simulink model "model"  (R2022b)
settings: Solver=VariableStepAuto  StartTime=0.0  StopTime=20  RelTol=1e-3
libraries: slpidlib x3, simulink x2, fuzblock x2, mpclib x1
settings Model: Creator=philf  LastModifiedBy=philf

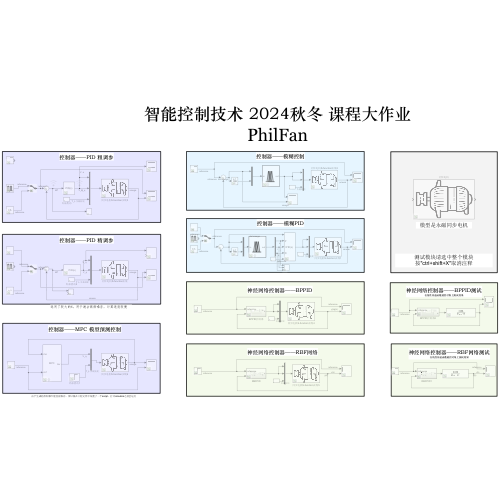
[thumbnail: Simulink's stored preview of the top-level diagram]
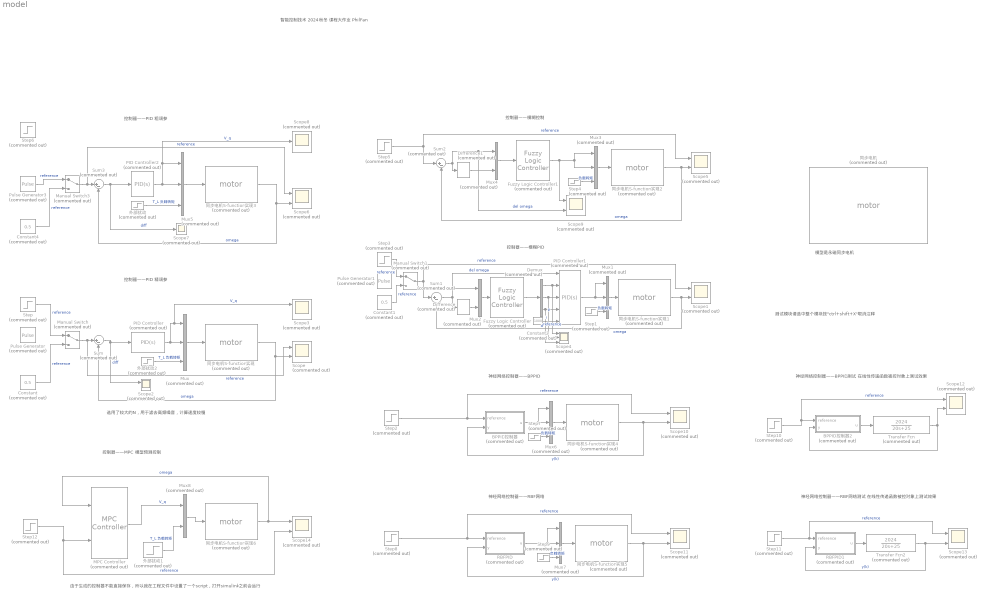
== system model ==
  note: 测试模块请选中整个模块按"ctrl+shift+X"取消注释
  note: 选用了较大的N，用于滤去高频噪音，计算速度较慢
  note: 控制器——PID 精调参
  note: 控制器——模糊PID
  note: 控制器——模糊控制
  note: 控制器——PID 粗调参
  note: 神经网络控制器——BPPID
  note: 神经网络控制器——RBF网络
  note: 神经网络控制器——BPPID测试
      | 在线性传递函数被控对象上测试效果
  note: 模型是永磁同步电机
  note: 神经网络控制器——RBF网络测试
      | 在线性传递函数被控对象上测试效果
  note: 控制器——MPC 模型预测控制
  note: 由于生成的控制器不能直接保存，所以我在工程文件中设置了一个script，打开simulink之前会运行
  note: 智能控制技术 2024秋冬 课程大作业
      | PhilFan
  BPPID控制器 : Subsystem  Commented=on
  BPPID控制器2 : Subsystem  Commented=on
  Constant : Constant  Commented=on  Value=0.5
  Constant1 : Constant  Commented=on  Value=0.5
  Constant2 : Constant  Commented=on  Value=1000
  Constant4 : Constant  Commented=on  Value=0.5
  Demux : Demux  Commented=on  Outputs=3
  Difference : simulink/Discrete/Difference  Commented=on  ICPrevInput=0.0  OutMin=[]  OutMax=[]  OutDataType=fixdt(1, 16)  OutScaling=2^-10  DoSatur=off
  Difference1 : simulink/Discrete/Difference  Commented=on  ICPrevInput=0.0  OutMin=[]  OutMax=[]  OutDataType=fixdt(1, 16)  OutScaling=2^-10  DoSatur=off
  Fuzzy Logic Controller : fuzblock/Fuzzy Logic  Controller  Commented=on  FIS='Fuzzy_PID2'  OutputSampleNumber=101  DataType=double  FuzzifiedInputs=off  RuleFiringStrengths=off  RuleOutputs=off  AggregatedOutputs=off  SimulateUsing=Interpreted execution  OutOfRangeInputValueMessage=warning  NoRuleFiredMessage=warning  EmptyOutputFuzzySetMessage=warning
  Fuzzy Logic Controller1 : fuzblock/Fuzzy Logic  Controller  Commented=on  FIS='Fuzzy_Control'  OutputSampleNumber=101  DataType=double  FuzzifiedInputs=off  RuleFiringStrengths=off  RuleOutputs=off  AggregatedOutputs=off  SimulateUsing=Interpreted execution  OutOfRangeInputValueMessage=warning  NoRuleFiredMessage=warning  EmptyOutputFuzzySetMessage=warning
  MPC Controller : mpclib/MPC Controller  Commented=on  SCDEnableBlockLinearizationSpecification=on  mpcobj=mpc1  is_multiple=0  enable_value=0  return_u0=off  updateMPCinCallerWorkspace=on  md_inport=off  mv_inport=off  uref_inport=off  return_cost=off  return_mvseq=off  return_qpstatus=off  return_xseq=off  return_state=off  return_ovseq=off  state_inport=off  umin_inport=off  umax_inport=off  ymin_inport=off  ymax_inport=off  cc_inport=off  ywt_inport=off  uwt_inport=off  duwt_inport=off  rhoeps_inport=off  pm_inport=off  MaximumP=10  HorizonChoice=FixedHorizon  n_ts=0.01  n_p=10  n_mv=2  n_md=0  n_ud=0  n_mo=1  n_uo=0  BlockDataType=double  SampleTimeInherited=off  switch_inport=off
  Manual Switch : ManualSwitch  Commented=on
  Manual Switch1 : ManualSwitch  Commented=on
  Manual Switch3 : ManualSwitch  Commented=on
  Mux{,1,3,5..7} (6 alike) : Mux  Commented=on  Inputs=3
  Mux2 : Mux  Commented=on  Inputs=2
  Mux4 : Mux  Commented=on  Inputs=2
  Mux8 : Mux  Commented=on  Inputs=[2 1]
  PID Controller : slpidlib/PID Controller  Commented=on  Controller=PID  Form=Parallel  TimeDomain=Continuous-time  UseExternalTs=off  SampleTime=-1  IntegratorMethod=Forward Euler  FilterMethod=Forward Euler  ControllerParametersSource=internal  P=2.82518808022121  I=29.1879779847918  UseKiTs=off  D=0.0345202590546222  N=158411.683957398  UseFilter=on  TunerSelectOption=Transfer Function Based (PID Tuner App)  InitialConditionSource=internal  InitialConditionForIntegrator=0  InitialConditionForFilter=0  DifferentiatorICPrevScaledInput=0  ExternalReset=none  TrackingMode=off  Kt=1  LimitOutput=off  SatLimitsSource=internal  UpperSaturationLimit=10  LowerSaturationLimit=-10  LinearizeAsGain=on  AntiWindupMode=none  Kb=1  LimitIntegrator=off  UpperIntegratorSaturationLimit=0.4  LowerIntegratorSaturationLimit=-0.4  POutMin=[]  POutMax=[]  IOutMin=[]  IOutMax=[]  DOutMin=[]  DOutMax=[]  NOutMin=[]  NOutMax=[]  SumOutMin=[]  SumOutMax=[]  SaturationOutMin=[]  SaturationOutMax=[]  PParamMin=[]  PParamMax=[]  IParamMin=[]  IParamMax=[]  DParamMin=[]  DParamMax=[]  NParamMin=[]  NParamMax=[]  KbParamMin=[]  KbParamMax=[]  KtParamMin=[]  KtParamMax=[]  KbOutMin=[]  KbOutMax=[]  KtOutMin=[]  KtOutMax=[]  IntegratorOutMin=[]  IntegratorOutMax=[]  FilterOutMin=[]  FilterOutMax=[]  SumI1OutMin=[]  SumI1OutMax=[]  SumI2OutMin=[]  SumI2OutMax=[]  SumI3OutMin=[]  SumI3OutMax=[]  SumI4OutMin=[]  SumI4OutMax=[]  SumDOutMin=[]  SumDOutMax=[]  DifferentiatorOutMin=[]  DifferentiatorOutMax=[]  FilterDiffOutCoefMin=[]  FilterDiffOutCoefMax=[]  ReciprocalOutMin=[]  ReciprocalOutMax=[]  SumDenOutMin=[]  SumDenOutMax=[]  SumNumOutMin=[]  SumNumOutMax=[]  DivideOutMin=[]  DivideOutMax=[]  UdiffTsProdOutMin=[]  UdiffTsProdOutMax=[]  NTsProdOutMin=[]  NTsProdOutMax=[]  UintegralTsProdOutMin=[]  UintegralTsProdOutMax=[]  UngainTsProdOutMin=[]  UngainTsProdOutMax=[]  ClampingZeroOutDataTypeStr=Inherit: Inherit via back propagation  ClampingZeroOutMin=[]  ClampingZeroOutMax=[]  FilterDenConstantOutDataTypeStr=Inherit: Inherit via back propagation  FilterDenConstantOutMin=[]  FilterDenConstantOutMax=[]  PCopyOutDataTypeStr=Inherit: Inherit via back propagation  PCopyOutMin=[]  PCopyOutMax=[]  NCopyOutDataTypeStr=Inherit: Inherit via back propagation  NCopyOutMin=[]  NCopyOutMax=[]  IntegratorContinuousStateAttributes=''  IntegratorStateMustResolveToSignalObject=off  IntegratorRTWStateStorageClass=Auto  FilterContinuousStateAttributes=''  FilterStateMustResolveToSignalObject=off  FilterRTWStateStorageClass=Auto  ParallelPVariant=InternalParameters  IdealPVariant=Disabled  IVariant=InternalParameters  DVariant=InternalParameters  IntegratorVariant=Continuous  SatVariant=Disabled  AWVariant=Passthrough  PCopyVariant=Disabled  TRVariant=Disabled  FdbkBlocksVariant=Forward  IdealPFdbkVariant=Disabled  SatFdbkVariant=Disabled  DerivativeFilterVariant=ContFilter  NVariant=InternalParameters  NCopyVariant=Disabled  FilterICVariant=InternalICsFilter  IntegratorICVariant=InternalICs  ExternalResetVariant=Disabled  TRSumVariant=Passthrough  SumFdbkVariant=Disabled  SumVariant=Sum_PID  TsampFilterVariant=InternalTs  TsampNgainVariant=Passthrough  TsampIntegralVariant=Passthrough  ExternalSaturationOutDataTypeStr=Inherit: Same as second input
  PID Controller1 : slpidlib/PID Controller  Commented=on  Controller=PID  Form=Parallel  TimeDomain=Continuous-time  UseExternalTs=off  SampleTime=-1  IntegratorMethod=Forward Euler  FilterMethod=Forward Euler  ControllerParametersSource=external  P=1  I=1  UseKiTs=off  D=0  N=100  UseFilter=on  TunerSelectOption=Transfer Function Based (PID Tuner App)  InitialConditionSource=internal  InitialConditionForIntegrator=0  InitialConditionForFilter=0  DifferentiatorICPrevScaledInput=0  ExternalReset=none  TrackingMode=off  Kt=1  LimitOutput=off  SatLimitsSource=internal  UpperSaturationLimit=inf  LowerSaturationLimit=-inf  LinearizeAsGain=on  AntiWindupMode=none  Kb=1  LimitIntegrator=off  UpperIntegratorSaturationLimit=inf  LowerIntegratorSaturationLimit=-inf  POutMin=[]  POutMax=[]  IOutMin=[]  IOutMax=[]  DOutMin=[]  DOutMax=[]  NOutMin=[]  NOutMax=[]  SumOutMin=[]  SumOutMax=[]  SaturationOutMin=[]  SaturationOutMax=[]  PParamMin=[]  PParamMax=[]  IParamMin=[]  IParamMax=[]  DParamMin=[]  DParamMax=[]  NParamMin=[]  NParamMax=[]  KbParamMin=[]  KbParamMax=[]  KtParamMin=[]  KtParamMax=[]  KbOutMin=[]  KbOutMax=[]  KtOutMin=[]  KtOutMax=[]  IntegratorOutMin=[]  IntegratorOutMax=[]  FilterOutMin=[]  FilterOutMax=[]  SumI1OutMin=[]  SumI1OutMax=[]  SumI2OutMin=[]  SumI2OutMax=[]  SumI3OutMin=[]  SumI3OutMax=[]  SumI4OutMin=[]  SumI4OutMax=[]  SumDOutMin=[]  SumDOutMax=[]  DifferentiatorOutMin=[]  DifferentiatorOutMax=[]  FilterDiffOutCoefMin=[]  FilterDiffOutCoefMax=[]  ReciprocalOutMin=[]  ReciprocalOutMax=[]  SumDenOutMin=[]  SumDenOutMax=[]  SumNumOutMin=[]  SumNumOutMax=[]  DivideOutMin=[]  DivideOutMax=[]  UdiffTsProdOutMin=[]  UdiffTsProdOutMax=[]  NTsProdOutMin=[]  NTsProdOutMax=[]  UintegralTsProdOutMin=[]  UintegralTsProdOutMax=[]  UngainTsProdOutMin=[]  UngainTsProdOutMax=[]  ClampingZeroOutDataTypeStr=Inherit: Inherit via back propagation  ClampingZeroOutMin=[]  ClampingZeroOutMax=[]  FilterDenConstantOutDataTypeStr=Inherit: Inherit via back propagation  FilterDenConstantOutMin=[]  FilterDenConstantOutMax=[]  PCopyOutDataTypeStr=Inherit: Inherit via back propagation  PCopyOutMin=[]  PCopyOutMax=[]  NCopyOutDataTypeStr=Inherit: Inherit via back propagation  NCopyOutMin=[]  NCopyOutMax=[]  IntegratorContinuousStateAttributes=''  IntegratorStateMustResolveToSignalObject=off  IntegratorRTWStateStorageClass=Auto  FilterContinuousStateAttributes=''  FilterStateMustResolveToSignalObject=off  FilterRTWStateStorageClass=Auto  ParallelPVariant=ExternalParameters  IdealPVariant=Disabled  IVariant=ExternalParameters  DVariant=ExternalParameters  IntegratorVariant=Continuous  SatVariant=Disabled  AWVariant=Passthrough  PCopyVariant=Disabled  TRVariant=Disabled  FdbkBlocksVariant=Forward  IdealPFdbkVariant=Disabled  SatFdbkVariant=Disabled  DerivativeFilterVariant=ContFilter  NVariant=ExternalParameters  NCopyVariant=Disabled  FilterICVariant=InternalICsFilter  IntegratorICVariant=InternalICs  ExternalResetVariant=Disabled  TRSumVariant=Passthrough  SumFdbkVariant=Disabled  SumVariant=Sum_PID  TsampFilterVariant=InternalTs  TsampNgainVariant=Passthrough  TsampIntegralVariant=Passthrough  ExternalSaturationOutDataTypeStr=Inherit: Same as second input
  PID Controller2 : slpidlib/PID Controller  Commented=on  Controller=PID  Form=Parallel  TimeDomain=Continuous-time  UseExternalTs=off  SampleTime=-1  IntegratorMethod=Forward Euler  FilterMethod=Forward Euler  ControllerParametersSource=internal  P=0.0095  I=0.5  UseKiTs=off  D=0.001  N=100  UseFilter=on  TunerSelectOption=Transfer Function Based (PID Tuner App)  InitialConditionSource=internal  InitialConditionForIntegrator=0  InitialConditionForFilter=0  DifferentiatorICPrevScaledInput=0  ExternalReset=none  TrackingMode=off  Kt=1  LimitOutput=off  SatLimitsSource=internal  UpperSaturationLimit=10  LowerSaturationLimit=-10  LinearizeAsGain=on  AntiWindupMode=none  Kb=1  LimitIntegrator=off  UpperIntegratorSaturationLimit=0.4  LowerIntegratorSaturationLimit=-0.4  POutMin=[]  POutMax=[]  IOutMin=[]  IOutMax=[]  DOutMin=[]  DOutMax=[]  NOutMin=[]  NOutMax=[]  SumOutMin=[]  SumOutMax=[]  SaturationOutMin=[]  SaturationOutMax=[]  PParamMin=[]  PParamMax=[]  IParamMin=[]  IParamMax=[]  DParamMin=[]  DParamMax=[]  NParamMin=[]  NParamMax=[]  KbParamMin=[]  KbParamMax=[]  KtParamMin=[]  KtParamMax=[]  KbOutMin=[]  KbOutMax=[]  KtOutMin=[]  KtOutMax=[]  IntegratorOutMin=[]  IntegratorOutMax=[]  FilterOutMin=[]  FilterOutMax=[]  SumI1OutMin=[]  SumI1OutMax=[]  SumI2OutMin=[]  SumI2OutMax=[]  SumI3OutMin=[]  SumI3OutMax=[]  SumI4OutMin=[]  SumI4OutMax=[]  SumDOutMin=[]  SumDOutMax=[]  DifferentiatorOutMin=[]  DifferentiatorOutMax=[]  FilterDiffOutCoefMin=[]  FilterDiffOutCoefMax=[]  ReciprocalOutMin=[]  ReciprocalOutMax=[]  SumDenOutMin=[]  SumDenOutMax=[]  SumNumOutMin=[]  SumNumOutMax=[]  DivideOutMin=[]  DivideOutMax=[]  UdiffTsProdOutMin=[]  UdiffTsProdOutMax=[]  NTsProdOutMin=[]  NTsProdOutMax=[]  UintegralTsProdOutMin=[]  UintegralTsProdOutMax=[]  UngainTsProdOutMin=[]  UngainTsProdOutMax=[]  ClampingZeroOutDataTypeStr=Inherit: Inherit via back propagation  ClampingZeroOutMin=[]  ClampingZeroOutMax=[]  FilterDenConstantOutDataTypeStr=Inherit: Inherit via back propagation  FilterDenConstantOutMin=[]  FilterDenConstantOutMax=[]  PCopyOutDataTypeStr=Inherit: Inherit via back propagation  PCopyOutMin=[]  PCopyOutMax=[]  NCopyOutDataTypeStr=Inherit: Inherit via back propagation  NCopyOutMin=[]  NCopyOutMax=[]  IntegratorContinuousStateAttributes=''  IntegratorStateMustResolveToSignalObject=off  IntegratorRTWStateStorageClass=Auto  FilterContinuousStateAttributes=''  FilterStateMustResolveToSignalObject=off  FilterRTWStateStorageClass=Auto  ParallelPVariant=InternalParameters  IdealPVariant=Disabled  IVariant=InternalParameters  DVariant=InternalParameters  IntegratorVariant=Continuous  SatVariant=Disabled  AWVariant=Passthrough  PCopyVariant=Disabled  TRVariant=Disabled  FdbkBlocksVariant=Forward  IdealPFdbkVariant=Disabled  SatFdbkVariant=Disabled  DerivativeFilterVariant=ContFilter  NVariant=InternalParameters  NCopyVariant=Disabled  FilterICVariant=InternalICsFilter  IntegratorICVariant=InternalICs  ExternalResetVariant=Disabled  TRSumVariant=Passthrough  SumFdbkVariant=Disabled  SumVariant=Sum_PID  TsampFilterVariant=InternalTs  TsampNgainVariant=Passthrough  TsampIntegralVariant=Passthrough  ExternalSaturationOutDataTypeStr=Inherit: Same as second input
  Pulse Generator : DiscretePulseGenerator  Commented=on  PulseType=Time based  Period=9  PulseWidth=50
  Pulse Generator1 : DiscretePulseGenerator  Commented=on  PulseType=Time based  Period=3.5  PulseWidth=50
  Pulse Generator3 : DiscretePulseGenerator  Commented=on  PulseType=Time based  Period=9  PulseWidth=50
  RBFPID : Subsystem  Commented=on
  RBFPID1 : Subsystem  Commented=on
  Scope{,1..3,5..6,9..14} (12 alike) : Scope  Commented=on  NumInputPorts=2
  Scope4 : Scope  Commented=on  NumInputPorts=3
  Scope7 : Scope  Commented=on
  Scope8 : Scope  Commented=on
  Step : Step  Commented=on  After=2  SampleTime=0
  Step{1,4,7,9} (4 alike) : Step  Commented=on  Time=4  After=0  SampleTime=0
  Step{2..3,6,8,10..12} (7 alike) : Step  Commented=on  SampleTime=0
  Step5 : Step  Commented=on  Time=0.2  SampleTime=0
  Sum{,1..3} (4 alike) : Sum  Commented=on  Inputs=|+-
  Transfer Fcn : TransferFcn  Commented=on  Numerator=[2024]  Denominator=[20 25]
  Transfer Fcn2 : TransferFcn  Commented=on  Numerator=[2024]  Denominator=[20 25]
  同步电机 : S-Function  Commented=on  FunctionName=motor  Parameters=R_s, L_d, L_q, psi_f, p, J, B  SFunctionDeploymentMode=off  EnableBusSupport=off  mask{R_s=0.01, L_d=0.001, L_q=0.0015, psi_f=0.1, p=4, J=0.01, B=0.001}
      mask prompts: R_s "定子电阻"; L_d "d 轴电感"; L_q "q 轴电感"; psi_f "永磁体磁链"; p "极对数"; J "转动惯量"; B "阻尼系数"
      mask DialogControl ParameterGroupVar Prompt: 参数
      mask Display: image('$imagefile'); % 使用工具条上的 "编辑图像" 进行更改。
  同步电机S-function实现 : S-Function  Commented=on  FunctionName=motor  Parameters=R_s, L_d, L_q, psi_f, p, J, B  SFunctionDeploymentMode=off  EnableBusSupport=off  mask{R_s=0.01, L_d=0.001, L_q=0.0015, psi_f=0.1, p=4, J=0.01, B=0.001}
      mask prompts: R_s "定子电阻"; L_d "d 轴电感"; L_q "q 轴电感"; psi_f "永磁体磁链"; p "极对数"; J "转动惯量"; B "阻尼系数"
      mask DialogControl ParameterGroupVar Prompt: 参数
      mask Display: image('$imagefile'); % 使用工具条上的 "编辑图像" 进行更改。
  同步电机S-function实现1 : S-Function  Commented=on  FunctionName=motor  Parameters=R_s, L_d, L_q, psi_f, p, J, B  SFunctionDeploymentMode=off  EnableBusSupport=off  mask{R_s=0.01, L_d=0.001, L_q=0.0015, psi_f=0.1, p=4, J=0.01, B=0.001}
      mask prompts: R_s "定子电阻"; L_d "d 轴电感"; L_q "q 轴电感"; psi_f "永磁体磁链"; p "极对数"; J "转动惯量"; B "阻尼系数"
      mask DialogControl ParameterGroupVar Prompt: 参数
      mask Display: image('$imagefile'); % 使用工具条上的 "编辑图像" 进行更改。
  同步电机S-function实现2 : S-Function  Commented=on  FunctionName=motor  Parameters=R_s, L_d, L_q, psi_f, p, J, B  SFunctionDeploymentMode=off  EnableBusSupport=off  mask{R_s=0.01, L_d=0.001, L_q=0.0015, psi_f=0.1, p=4, J=0.01, B=0.001}
      mask prompts: R_s "定子电阻"; L_d "d 轴电感"; L_q "q 轴电感"; psi_f "永磁体磁链"; p "极对数"; J "转动惯量"; B "阻尼系数"
      mask DialogControl ParameterGroupVar Prompt: 参数
      mask Display: image('$imagefile'); % 使用工具条上的 "编辑图像" 进行更改。
  同步电机S-function实现3 : S-Function  Commented=on  FunctionName=motor  Parameters=R_s, L_d, L_q, psi_f, p, J, B  SFunctionDeploymentMode=off  EnableBusSupport=off  mask{R_s=0.01, L_d=0.001, L_q=0.0015, psi_f=0.1, p=4, J=0.01, B=0.001}
      mask prompts: R_s "定子电阻"; L_d "d 轴电感"; L_q "q 轴电感"; psi_f "永磁体磁链"; p "极对数"; J "转动惯量"; B "阻尼系数"
      mask DialogControl ParameterGroupVar Prompt: 参数
      mask Display: image('$imagefile'); % 使用工具条上的 "编辑图像" 进行更改。
  同步电机S-function实现4 : S-Function  Commented=on  FunctionName=motor  Parameters=R_s, L_d, L_q, psi_f, p, J, B  SFunctionDeploymentMode=off  EnableBusSupport=off  mask{R_s=0.01, L_d=0.001, L_q=0.0015, psi_f=0.1, p=4, J=0.01, B=0.001}
      mask prompts: R_s "定子电阻"; L_d "d 轴电感"; L_q "q 轴电感"; psi_f "永磁体磁链"; p "极对数"; J "转动惯量"; B "阻尼系数"
      mask DialogControl ParameterGroupVar Prompt: 参数
      mask Display: image('$imagefile'); % 使用工具条上的 "编辑图像" 进行更改。
  同步电机S-function实现5 : S-Function  Commented=on  FunctionName=motor  Parameters=R_s, L_d, L_q, psi_f, p, J, B  SFunctionDeploymentMode=off  EnableBusSupport=off  mask{R_s=0.01, L_d=0.001, L_q=0.0015, psi_f=0.1, p=4, J=0.01, B=0.001}
      mask prompts: R_s "定子电阻"; L_d "d 轴电感"; L_q "q 轴电感"; psi_f "永磁体磁链"; p "极对数"; J "转动惯量"; B "阻尼系数"
      mask DialogControl ParameterGroupVar Prompt: 参数
      mask Display: image('$imagefile'); % 使用工具条上的 "编辑图像" 进行更改。
  同步电机S-function实现6 : S-Function  Commented=on  FunctionName=motor  Parameters=R_s, L_d, L_q, psi_f, p, J, B  SFunctionDeploymentMode=off  EnableBusSupport=off  mask{R_s=0.01, L_d=0.001, L_q=0.0015, psi_f=0.1, p=4, J=0.01, B=0.001}
      mask prompts: R_s "定子电阻"; L_d "d 轴电感"; L_q "q 轴电感"; psi_f "永磁体磁链"; p "极对数"; J "转动惯量"; B "阻尼系数"
      mask DialogControl ParameterGroupVar Prompt: 参数
      mask Display: image('$imagefile'); % 使用工具条上的 "编辑图像" 进行更改。
  外部扰动 : Step  Commented=on  Time=4  After=0  SampleTime=0
  外部扰动1 : Step  Commented=on  Time=4  After=0  SampleTime=0
  外部扰动2 : Step  Commented=on  Time=4  After=0  SampleTime=0
  wires:
  同步电机S-function实现/1 -> Sum/2, Scope/2  "omega"
  Mux/1 -> 同步电机S-function实现/1
  外部扰动2/1 -> Mux/3  "T_L 负载转矩"
  Manual Switch/1 -> Scope/1, Sum/1  "reference"
  Sum/1 -> PID Controller/1, Scope2/1  "diff"
  PID Controller/1 -> Scope3/1, Mux/1, Mux/2  "V_q"
  Step/1 -> Manual Switch/1  "reference"
  Constant/1 -> Manual Switch/2  "reference"
  Constant1/1 -> Manual Switch1/2  "reference"
  Manual Switch1/1 -> Scope1/1, Sum1/1  "reference"
  Step3/1 -> Manual Switch1/1  "reference"
  Step1/1 -> Mux1/3  "负载转矩"
  Mux1/1 -> 同步电机S-function实现1/1
  同步电机S-function实现1/1 -> Sum1/2, Scope1/2  "omega"
  Difference/1 -> Mux2/2
  Demux/1 -> Scope4/1, PID Controller1/2  "p"
  Demux/2 -> Scope4/2, PID Controller1/3  "i"
  Mux2/1 -> Fuzzy Logic Controller/1
  Fuzzy Logic Controller/1 -> Demux/1
  PID Controller1/1 -> Mux1/1, Mux1/2
  Sum1/1 -> PID Controller1/1, Mux2/1, Difference/1  "del omega"
  Demux/3 -> Scope4/3, PID Controller1/4  "d"
  Constant2/1 -> PID Controller1/5  "reference"
  Sum2/1 -> Scope9/2, Mux4/1, Difference1/1  "del omega"
  Mux4/1 -> Fuzzy Logic Controller1/1
  Difference1/1 -> Mux4/2
  Fuzzy Logic Controller1/1 -> Scope9/1, Mux3/2, Mux3/1
  Step5/1 -> Sum2/1, Scope5/1  "reference"
  Mux3/1 -> 同步电机S-function实现2/1
  Step4/1 -> Mux3/3  "负载转矩"
  同步电机S-function实现2/1 -> Sum2/2, Scope5/2  "omega"
  Pulse Generator3/1 -> Manual Switch3/1  "reference"
  Manual Switch3/1 -> Scope6/1, Sum3/1  "reference"
  Sum3/1 -> Scope7/1, PID Controller2/1  "diff"
  外部扰动/1 -> Mux5/3  "T_L 负载转矩"
  PID Controller2/1 -> Mux5/2, Mux5/1, Scope8/1  "V_q"
  Constant4/1 -> Manual Switch3/2  "reference"
  Mux5/1 -> 同步电机S-function实现3/1
  同步电机S-function实现3/1 -> Sum3/2, Scope6/2  "omega"
  BPPID控制器/1(u) -> Mux6/2, Mux6/1
  Step7/1 -> Mux6/3  "负载转矩"
  同步电机S-function实现4/1 -> BPPID控制器/2(y), Scope10/2  "y(k)"
  Step2/1 -> BPPID控制器/1(reference), Scope10/1  "reference"
  同步电机S-function实现5/1 -> Scope11/2, RBFPID/2(y)  "y(k)"
  Step8/1 -> RBFPID/1(reference), Scope11/1  "reference"
  BPPID控制器2/1(u) -> Transfer Fcn/1
  Transfer Fcn/1 -> Scope12/2, BPPID控制器2/2(y)
  Step10/1 -> Scope12/1, BPPID控制器2/1(reference)  "reference"
  RBFPID/1(u) -> Mux7/1, Mux7/2
  Mux7/1 -> 同步电机S-function实现5/1
  Step9/1 -> Mux7/3  "负载转矩"
  Step11/1 -> RBFPID1/1(reference), Scope13/1  "reference"
  Transfer Fcn2/1 -> Scope13/2, RBFPID1/2(y)  "y(k)"
  RBFPID1/1(u) -> Transfer Fcn2/1
  Step12/1 -> Scope14/2, MPC Controller/2  "reference"
  外部扰动1/1 -> Mux8/2  "T_L 负载转矩"
  同步电机S-function实现6/1 -> MPC Controller/1, Scope14/1  "omega"
  Mux8/1 -> 同步电机S-function实现6/1
  MPC Controller/1 -> Mux8/1  "V_q"
  Mux6/1 -> 同步电机S-function实现4/1

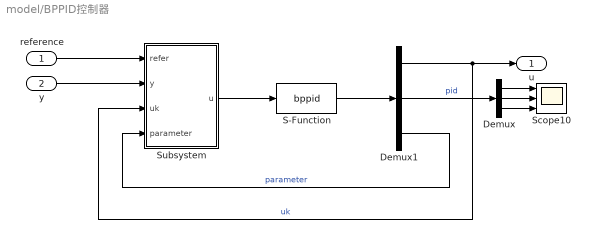
== system model/BPPID控制器 ==
  reference : Inport
  y : Inport  Port=2
  Demux : Demux  Outputs=3
  Demux1 : Demux  Outputs=[1 3 48]
  S-Function : S-Function  FunctionName=bppid  Parameters=T,nh,xite,alfa  SFunctionDeploymentMode=off  EnableBusSupport=off  mask{T=0.01, nh=8, xite=0.03, alfa=0.3}
      mask DialogControl ParameterGroupVar Prompt: 参数
  Scope10 : Scope  NumInputPorts=3
  Subsystem : Subsystem
  u : Outport
  wires:
  Demux1/1 -> u/1, Subsystem/3(uk)  "uk"
  Demux1/2 -> Demux/1  "pid"
  S-Function/1 -> Demux1/1
  reference/1 -> Subsystem/1(refer)
  y/1 -> Subsystem/2(y)
  Demux1/3 -> Subsystem/4(parameter)  "parameter"
  Subsystem/1(u) -> S-Function/1
  Demux/1 -> Scope10/1
  Demux/2 -> Scope10/2
  Demux/3 -> Scope10/3

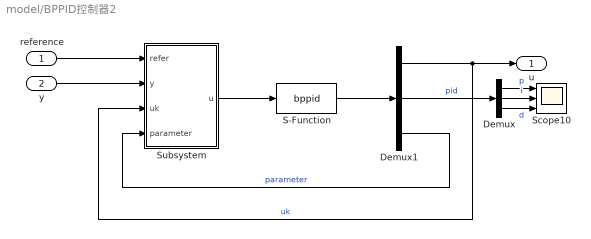
== system model/BPPID控制器2 ==
  reference : Inport
  y : Inport  Port=2
  Demux : Demux  Outputs=3
  Demux1 : Demux  Outputs=[1 3 48]
  S-Function : S-Function  FunctionName=bppid  Parameters=T,nh,xite,alfa  SFunctionDeploymentMode=off  EnableBusSupport=off  mask{T=0.01, nh=8, xite=0.03, alfa=0.3}
      mask DialogControl ParameterGroupVar Prompt: 参数
  Scope10 : Scope  NumInputPorts=3
  Subsystem : Subsystem
  u : Outport
  wires:
  Demux1/1 -> u/1, Subsystem/3(uk)  "uk"
  Demux1/2 -> Demux/1  "pid"
  S-Function/1 -> Demux1/1
  reference/1 -> Subsystem/1(refer)
  y/1 -> Subsystem/2(y)
  Demux1/3 -> Subsystem/4(parameter)  "parameter"
  Subsystem/1(u) -> S-Function/1
  Demux/1 -> Scope10/1  "p"
  Demux/2 -> Scope10/2  "i"
  Demux/3 -> Scope10/3  "d"

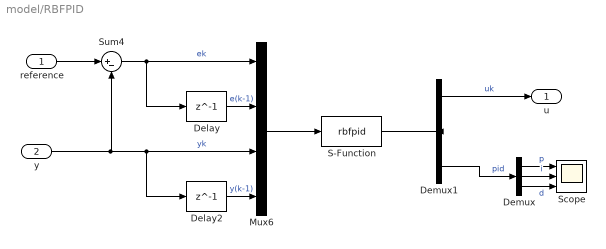
== system model/RBFPID ==
  reference : Inport
  y : Inport  Port=2
  Delay : Delay  DelayLength=1  InitialCondition=0
  Delay2 : Delay  DelayLength=1  InitialCondition=0
  Demux : Demux  Outputs=3
  Demux1 : Demux  Outputs=[1 1 3]
  Mux6 : Mux
  S-Function : S-Function  FunctionName=rbfpid  SFunctionDeploymentMode=off  EnableBusSupport=off
      mask DialogControl ParameterGroupVar Prompt: 参数
  Scope : Scope  NumInputPorts=3
  Sum4 : Sum  Inputs=|+-
  u : Outport
  wires:
  Demux1/1 -> u/1  "uk"
  S-Function/1 -> Demux1/1
  Mux6/1 -> S-Function/1
  Sum4/1 -> Delay/1, Mux6/1  "ek"
  Delay2/1 -> Mux6/4  "y(k-1)"
  reference/1 -> Sum4/1
  Delay/1 -> Mux6/2  "e(k-1)"
  y/1 -> Mux6/3, Delay2/1, Sum4/2  "yk"
  Demux1/3 -> Demux/1  "pid"
  Demux/1 -> Scope/1  "p"
  Demux/2 -> Scope/2  "i"
  Demux/3 -> Scope/3  "d"

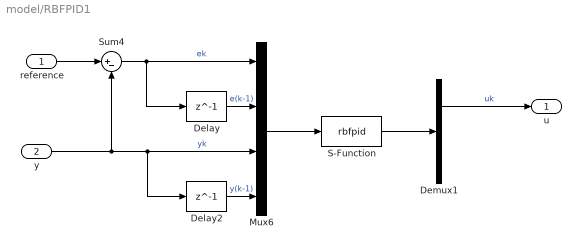
== system model/RBFPID1 ==
  reference : Inport
  y : Inport  Port=2
  Delay : Delay  DelayLength=1  InitialCondition=0
  Delay2 : Delay  DelayLength=1  InitialCondition=0
  Demux1 : Demux  Outputs=2
  Mux6 : Mux
  S-Function : S-Function  FunctionName=rbfpid  SFunctionDeploymentMode=off  EnableBusSupport=off
      mask DialogControl ParameterGroupVar Prompt: 参数
  Sum4 : Sum  Inputs=|+-
  u : Outport
  wires:
  Demux1/1 -> u/1  "uk"
  S-Function/1 -> Demux1/1
  Mux6/1 -> S-Function/1
  Sum4/1 -> Delay/1, Mux6/1  "ek"
  Delay2/1 -> Mux6/4  "y(k-1)"
  reference/1 -> Sum4/1
  Delay/1 -> Mux6/2  "e(k-1)"
  y/1 -> Mux6/3, Delay2/1, Sum4/2  "yk"

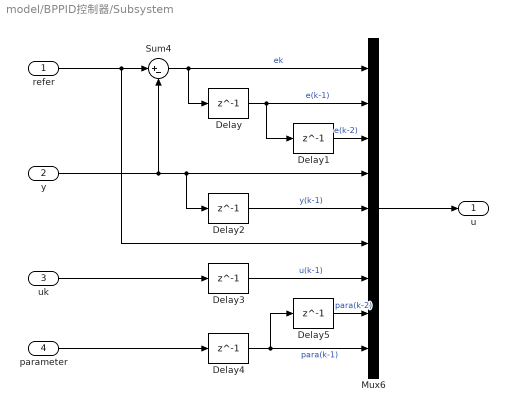
== system model/BPPID控制器/Subsystem ==
  refer : Inport
  y : Inport  Port=2
  uk : Inport  Port=3
  parameter : Inport  Port=4
  Delay{,1..5} (6 alike) : Delay  DelayLength=1  InitialCondition=0
  Mux6 : Mux  Inputs=9
  Sum4 : Sum  Inputs=|+-
  u : Outport
  wires:
  parameter/1 -> Delay4/1
  y/1 -> Sum4/2, Delay2/1, Mux6/4
  Delay3/1 -> Mux6/7  "u(k-1)"
  Delay4/1 -> Delay5/1, Mux6/9  "para(k-1)"
  Delay/1 -> Delay1/1, Mux6/2  "e(k-1)"
  refer/1 -> Mux6/6, Sum4/1
  Delay5/1 -> Mux6/8  "para(k-2)"
  Delay1/1 -> Mux6/3  "e(k-2)"
  Delay2/1 -> Mux6/5  "y(k-1)"
  Sum4/1 -> Mux6/1, Delay/1  "ek"
  uk/1 -> Delay3/1
  Mux6/1 -> u/1

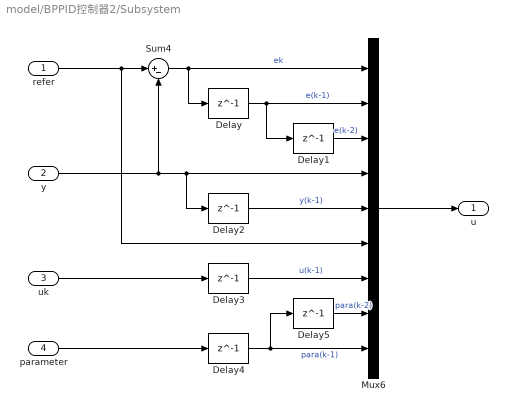
== system model/BPPID控制器2/Subsystem ==
  refer : Inport
  y : Inport  Port=2
  uk : Inport  Port=3
  parameter : Inport  Port=4
  Delay{,1..5} (6 alike) : Delay  DelayLength=1  InitialCondition=0
  Mux6 : Mux  Inputs=9
  Sum4 : Sum  Inputs=|+-
  u : Outport
  wires:
  parameter/1 -> Delay4/1
  y/1 -> Sum4/2, Delay2/1, Mux6/4
  Delay3/1 -> Mux6/7  "u(k-1)"
  Delay4/1 -> Delay5/1, Mux6/9  "para(k-1)"
  Delay/1 -> Delay1/1, Mux6/2  "e(k-1)"
  refer/1 -> Mux6/6, Sum4/1
  Delay5/1 -> Mux6/8  "para(k-2)"
  Delay1/1 -> Mux6/3  "e(k-2)"
  Delay2/1 -> Mux6/5  "y(k-1)"
  Sum4/1 -> Mux6/1, Delay/1  "ek"
  uk/1 -> Delay3/1
  Mux6/1 -> u/1
